simulink model "Assignment"  (R2021b)
settings: Solver=ode45  StartTime=0.0  StopTime=tsimul  MaxStep=.1e-3  RelTol=1e-3
values from neighbouring files (symbols this model uses):
  A = pi*R_turbine^2    (= 4536.45979178)    [ref.m]
  cp = max(0,c1*(c2*k1-c3*angle_pitch-c4*angle_pitch^c5-c6).*exp(-c7*k1))    [ref.m]
  f = 47    [ref.m]
  Jtot = 9e6    (= 9000000)    [ref.m]
  n_multiplier = 80    [ref.m]
  Pnom = 2e6    (= 2000000)    [ref.m]
  R_turbine = 38    [ref.m]
  rho = 1.225    [ref.m]
  Rr = 0.009    [ref.m]
  Rs = 0.005    [ref.m]
  tsr = 0:.1:17    [ref.m]
  Vnom = 960    [ref.m]
  w_ini = 2*pi*25/80    (= 1.96349540849)    [ref.m]
  w_speed = 14    [ref.m]
  wg = 2*pi*f/pols    (= 147.654854719)    [ref.m]
  Xm = 2*pi*f*15E-3    (= 4.42964564156)    [ref.m]
  Xr = 2*pi*f*3E-4    (= 0.0885929128312)    [ref.m]
  Xs = 2*pi*f*4e-4    (= 0.118123883775)    [ref.m]
libraries: spsAsynchronousMachineSIUnitsLib x1, spsGroundLib x1, spsPower3phInstantaneousLib x1, spsRMSLib x1, spsThreePhaseProgrammableVoltageSourceLib x1, spsThreePhaseVIMeasurementLib x1, spspowerguiLib x1
settings Model: Creator=santi  LastModifiedBy=santi

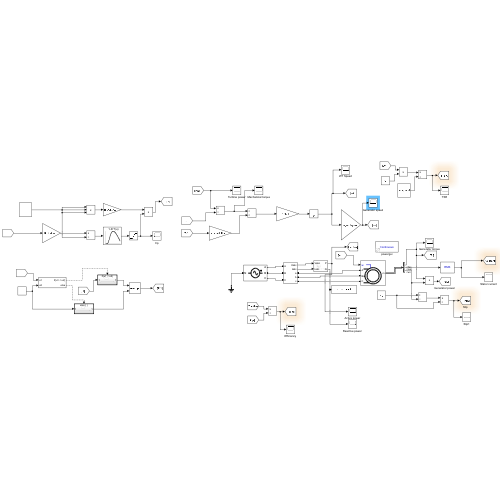
[thumbnail: Simulink's stored preview of the top-level diagram]
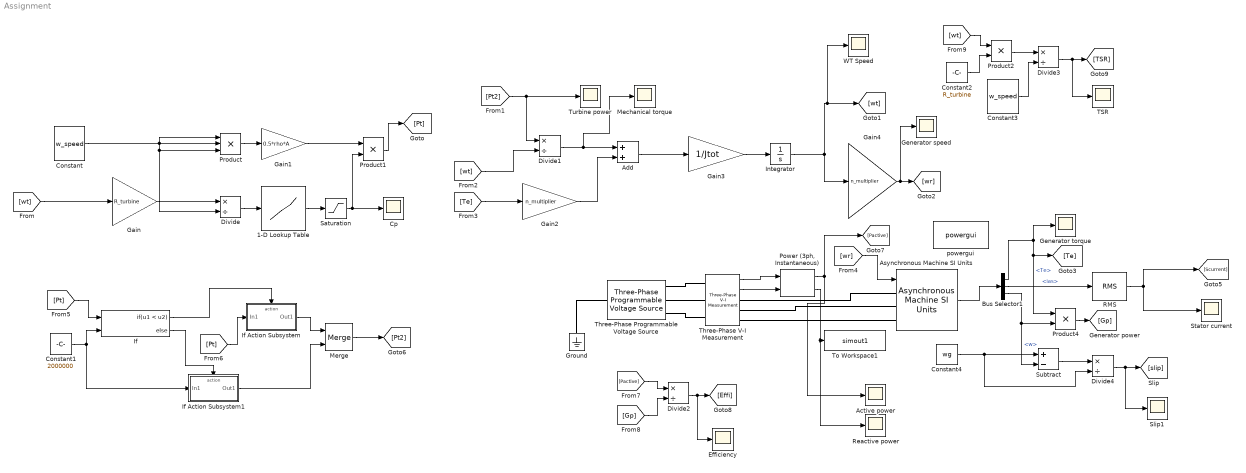
== system Assignment ==
  1-D Lookup Table : Lookup_n-D  NumberOfTableDimensions=1  BreakpointsForDimension1=tsr  Table=cp  InternalRulePriority=Speed  RndMeth=Simplest  InputSameDT=on
  Active power : Scope
  Add : Sum
  Asynchronous Machine SI Units : spsAsynchronousMachineSIUnitsLib/Asynchronous Machine SI Units  RotorType=Squirrel-cage  PresetModel=No  MechanicalLoad=Speed w  ShowDetailedParameters=on  ReferenceFrame=Rotor  Units=SI  MeasurementBus=on  NominalParameters=[Pnom Vnom f]  VoltageRatio=1  Stator=[Rs Xs/(2*pi*f)]  Rotor=[Rr Xr/(2*pi*f)]  Cage1=[0.4155 0.002066]  Cage2=[0.4168 0.0003495]  Lm=Xm/(2*pi*f)  Mechanical=[0.05 0.005879 2]  PolePairs=pols  InitialConditions=[0.01 0 0 0 0 0 0 0]  SimulateSaturation=off  Saturation=[14.03593122, 27.81365428, 53.79336849, 72.68890987, 97.98006896, 148.6815601, 215.7428561, 302.9841135, 428.7778367 ; 230, 322, 414, 460, 506, 552, 598, 644, 690]  LoadFlowParameters=1492000  TsPowergui=0  TsBlock=-1  IterativeModel=Trapezoidal non iterative  IterativeDiscreteModel=Trapezoidal non iterative  Pmec=1.492e+006
  Bus Selector1 : BusSelector  OutputSignals=Te,ias,w
  Constant : Constant  Value=w_speed
  Constant1 : Constant  Value=2000000
  Constant2 : Constant  Value=R_turbine
  Constant3 : Constant  Value=w_speed
  Constant4 : Constant  Value=wg
  Cp : Scope
  Divide{,1..4} (5 alike) : Product  Inputs=*/
  Efficiency : Scope
  Gain : Gain  Gain=R_turbine
  Gain1 : Gain  Gain=0.5*rho*A
  Gain2 : Gain  Gain=n_multiplier
  Gain3 : Gain  Gain=1/Jtot
  Gain4 : Gain  Gain=n_multiplier
  Generator speed : Scope
  Generator torque : Scope
  Ground : spsGroundLib/Ground  LConnTagsString=a
  If : If  NumInputs=2  IfExpression=u1 < u2
  If Action Subsystem : Subsystem  TreatAsAtomicUnit=on
  If Action Subsystem1 : Subsystem  TreatAsAtomicUnit=on
  Integrator : Integrator  InitialCondition=w_ini
  Mechanical torque : Scope
  Merge : Merge
  "Power (3ph, Instantaneous)" : spsPower3phInstantaneousLib/Power (3ph, Instantaneous)
  Product : Product  Inputs=3
  Product1 : Product
  Product2 : Product
  Product4 : Product
  RMS : spsRMSLib/RMS  TrueRMS=on  Freq=60  RMSInit=120  Ts=0
  Reactive power : Scope
  Saturation : Saturate  UpperLimit=1  LowerLimit=0
  Slip1 : Scope
  Stator current : Scope
  Subtract : Sum  Inputs=+-
  TSR : Scope
  Three-Phase Programmable Voltage Source : spsThreePhaseProgrammableVoltageSourceLib/Three-Phase Programmable Voltage Source  PositiveSequence="[Vnom  0 f]"  VariationEntity=None  VariationType=Table of time-amplitude pairs  VariationTypeAlt=Step  VariationStep=0.5  VariationRate=10  VariationMagnitude=0.3  VariationFrequency=2  VariationTiming=[1 2]  VariationPhaseA=off  Amplitudes=[1 0.8 1.2 1.0]  TimeValues=[0 0.1 0.15 0.2]  HarmonicGeneration=off  HarmonicA=[3 0.2 -25 0]  HarmonicB=[2 0.15 35 2]  Timing="[0.05  3]"  BusType=swing  Pref=0  Qref=0  Qmin=-inf  Qmax=inf
  Three-Phase V-I Measurement : spsThreePhaseVIMeasurementLib/Three-Phase V-I Measurement  VoltageMeasurement=phase-to-ground  SetLabelV=off  LabelV=Vabc  Vpu=off  VpuLL=off  CurrentMeasurement=yes  SetLabelI=off  LabelI=Iabc  Ipu=off  Pbase=100e6  Vbase=500e3  OutputType=Complex  PhasorSimulation=off  PSBequivalent=0
  To Workspace1 : ToWorkspace  VariableName=simout1  SaveFormat=Timeseries  SampleTime=-1
  Turbine power : Scope
  WT Speed : Scope
  powergui : spspowerguiLib/powergui  Priority=1  SimulationMode=Continuous  SampleTime=50e-6  frequency=60  Iterations=50  frequencyindice=47  Pbase=100e6  ErrMax=1e-4  UnitsV=kV  UnitsW=MW  buscounter=0  FunctionMessages=off  echomessages=off  EnableUseOfTLC=off  CurrentSourceSwitches=off  DisableSnubberDevices=off  DisableRonSwitches=off  DisableVfSwitches=off  DisplayEquations=off  AutomaticDiscreteSolvers=off  SolverType=Tustin/Backward Euler (TBE)  Interpol=off  ExternalGateDelay=off  methode=off  Ts=100  x0status=blocks  SPID=on  SwTol=0  HookPort=off  NonlinearTolerance=1e-4  nMaxIteration=100  ContinueOnMaxIteration=off  RestoreLinks=warning  ResistiveCurrentMeasurement=off  Frange=[0:2:500]  Ylog=off  Xlog=on  ShowGrid=off  save=off  variable=ZData  structure=0  ZoomFFT=off  StartTime=0.0  cycles=1  DisplayStyle=1  fundamental=60  FreqAxis=off  MaxFrequency=1000  frequencyindicesteady=1  RmsSteady=1  display=off
  wires:
  [wt] -> Gain/1
  Constant/1 -> Product/1, Product/3, Divide/2, Product/2
  Gain/1 -> Divide/1
  Product/1 -> Gain1/1
  Divide/1 -> 1-D Lookup Table/1
  1-D Lookup Table/1 -> Saturation/1
  Gain1/1 -> Product1/1
  Saturation/1 -> Cp/1, Product1/2
  Product1/1 -> [Pt]
  [wt] -> Divide1/2
  Divide1/1 -> Mechanical torque/1, Add/1
  Gain2/1 -> Add/2
  [Te] -> Gain2/1
  Add/1 -> Gain3/1
  Gain3/1 -> Integrator/1
  Integrator/1 -> Gain4/1, WT Speed/1, [wt]
  Gain4/1 -> Generator speed/1, [wr]
  Three-Phase V-I Measurement/1 -> "Power (3ph, Instantaneous)"/1
  Three-Phase V-I Measurement/2 -> "Power (3ph, Instantaneous)"/2
  [wr] -> Asynchronous Machine SI Units/1
  Bus Selector1/1 -> Product4/1, [Te], Generator torque/1  "<Te>"
  "Power (3ph, Instantaneous)"/1 -> [Pactive], Active power/1
  "Power (3ph, Instantaneous)"/2 -> Reactive power/1, To Workspace1/1
  [Pt2] -> Divide1/1, Turbine power/1
  Asynchronous Machine SI Units/1 -> Bus Selector1/1
  Bus Selector1/3 -> Product4/2, Subtract/2  "<w>"
  Bus Selector1/2 -> RMS/1  "<ias>"
  [Pt] -> If/1
  Constant1/1 -> If Action Subsystem1/1(In1), If/2
  If/1 -> If Action Subsystem/Action
  [Pt] -> If Action Subsystem/1(In1)
  If/2 -> If Action Subsystem1/Action
  If Action Subsystem/1(Out1) -> Merge/1
  If Action Subsystem1/1(Out1) -> Merge/2
  Merge/1 -> [Pt2]
  RMS/1 -> Stator current/1, [Scurrent]
  [Pactive] -> Divide2/1
  [Gp] -> Divide2/2
  Divide2/1 -> Efficiency/1, [Effi]
  [wt] -> Product2/1
  Constant2/1 -> Product2/2
  Product2/1 -> Divide3/1
  Constant3/1 -> Divide3/2
  Divide3/1 -> TSR/1, [TSR]
  Constant4/1 -> Divide4/2, Subtract/1
  Subtract/1 -> Divide4/1
  Divide4/1 -> Slip1/1, [slip]
  Product4/1 -> [Gp]
  connections:
  Ground/LConn1 -- Three-Phase Programmable Voltage Source/LConn1
  Three-Phase Programmable Voltage Source/RConn1 -- Three-Phase V-I Measurement/LConn1
  Three-Phase Programmable Voltage Source/RConn2 -- Three-Phase V-I Measurement/LConn2
  Three-Phase Programmable Voltage Source/RConn3 -- Three-Phase V-I Measurement/LConn3
  Asynchronous Machine SI Units/LConn1 -- Three-Phase V-I Measurement/RConn1
  Asynchronous Machine SI Units/LConn2 -- Three-Phase V-I Measurement/RConn2
  Asynchronous Machine SI Units/LConn3 -- Three-Phase V-I Measurement/RConn3

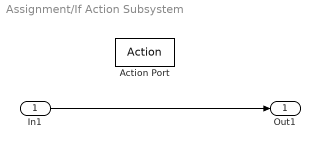
== system Assignment/If Action Subsystem ==
  In1 : Inport
  Action Port : ActionPort  ActionPortLabel=if(u1 < u2)
  Out1 : Outport
  wires:
  In1/1 -> Out1/1

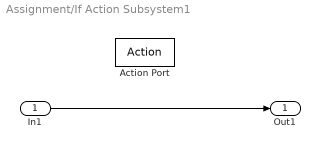
== system Assignment/If Action Subsystem1 ==
  In1 : Inport
  Action Port : ActionPort  ActionPortLabel=else
  Out1 : Outport
  wires:
  In1/1 -> Out1/1
